simulink model "P8lototoV3p2b"  (R2020b)
settings: Solver=ode5  StartTime=0.0  StopTime=inf  RelTol=1e-3
undefined symbols (not defined in the file): National_Instruments, PCI
libraries: sldrtlib x2, cstblocks x2, simulink x2, pid_lib x1
settings Model: SimulationMode=external  Creator=Usuario_UMA  LastModifiedBy=alumnoic03
settings RTWCC: Description=Simulink Desktop Real-Time  SystemTargetFile=sldrt.tlc  TemplateMakefile=sldrt.tmf  RTWCompilerOptimization=on
settings CodeAppCC: MaxIdLength=95
settings SimulinkDesktopRealTimeCC: TargetPreCompLibLocation=C:\Program Files\MATLAB\R2020\toolbox\sldrt\lib\win64

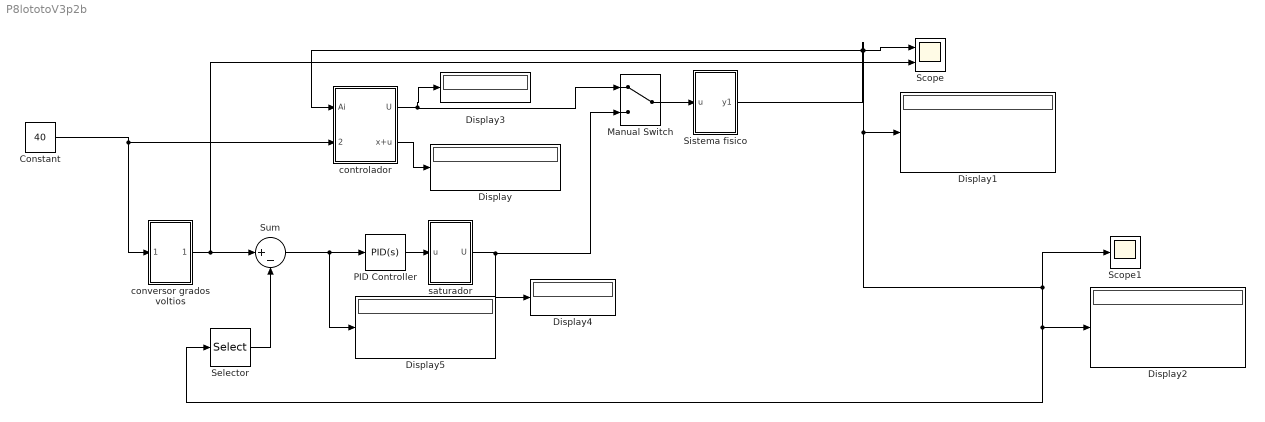
== system P8lototoV3p2b ==
  Constant : Constant  Value=40
  Display{,1..5} (6 alike) : Display
  Manual Switch : ManualSwitch
  PID Controller : pid_lib/PID Controller  Controller=PID  Form=Parallel  TimeDomain=Continuous-time  UseExternalTs=off  SampleTime=-1  IntegratorMethod=Forward Euler  FilterMethod=Forward Euler  ControllerParametersSource=internal  P=1.17  I=1.96  D=0.118  UseFilter=on  N=100  TunerSelectOption=Transfer Function Based (PID Tuner App)  InitialConditionSource=internal  InitialConditionForIntegrator=0  InitialConditionForFilter=0  DifferentiatorICPrevScaledInput=0  ExternalReset=none  TrackingMode=off  Kt=1  LimitOutput=off  SatLimitsSource=internal  UpperSaturationLimit=inf  LowerSaturationLimit=-inf  LinearizeAsGain=on  AntiWindupMode=none  Kb=1  POutMin=[]  POutMax=[]  IOutMin=[]  IOutMax=[]  DOutMin=[]  DOutMax=[]  NOutMin=[]  NOutMax=[]  SumOutMin=[]  SumOutMax=[]  SaturationOutMin=[]  SaturationOutMax=[]  PParamMin=[]  PParamMax=[]  IParamMin=[]  IParamMax=[]  DParamMin=[]  DParamMax=[]  NParamMin=[]  NParamMax=[]  KbParamMin=[]  KbParamMax=[]  KtParamMin=[]  KtParamMax=[]  KbOutMin=[]  KbOutMax=[]  KtOutMin=[]  KtOutMax=[]  IntegratorOutMin=[]  IntegratorOutMax=[]  FilterOutMin=[]  FilterOutMax=[]  SumI1OutMin=[]  SumI1OutMax=[]  SumI2OutMin=[]  SumI2OutMax=[]  SumI3OutMin=[]  SumI3OutMax=[]  SumI4OutMin=[]  SumI4OutMax=[]  SumDOutMin=[]  SumDOutMax=[]  DifferentiatorOutMin=[]  DifferentiatorOutMax=[]  FilterDiffOutCoefMin=[]  FilterDiffOutCoefMax=[]  ReciprocalOutMin=[]  ReciprocalOutMax=[]  SumDenOutMin=[]  SumDenOutMax=[]  SumNumOutMin=[]  SumNumOutMax=[]  DivideOutMin=[]  DivideOutMax=[]  UdiffTsProdOutMin=[]  UdiffTsProdOutMax=[]  NTsProdOutMin=[]  NTsProdOutMax=[]  UintegralTsProdOutMin=[]  UintegralTsProdOutMax=[]  UngainTsProdOutMin=[]  UngainTsProdOutMax=[]  IntegratorContinuousStateAttributes=''  IntegratorStateMustResolveToSignalObject=off  IntegratorRTWStateStorageClass=Auto  FilterContinuousStateAttributes=''  FilterStateMustResolveToSignalObject=off  FilterRTWStateStorageClass=Auto  ParallelPVariant=InternalParameters  IdealPVariant=Disabled  IVariant=InternalParameters  DVariant=InternalParameters  IntegratorVariant=Continuous  SatVariant=Disabled  AWVariant=Passthrough  PCopyVariant=Disabled  TRVariant=Disabled  FdbkBlocksVariant=Forward  IdealPFdbkVariant=Disabled  SatFdbkVariant=Disabled  DerivativeFilterVariant=ContFilter  NVariant=InternalParameters  NCopyVariant=Disabled  FilterICVariant=InternalICsFilter  IntegratorICVariant=InternalICs  ExternalResetVariant=Disabled  TRSumVariant=Passthrough  SumFdbkVariant=Disabled  SumVariant=Sum_PID  TsampFilterVariant=InternalTs  TsampNgainVariant=Passthrough  TsampIntegralVariant=Passthrough  ExternalSaturationOutDataTypeStr=Inherit: Same as second input
  Scope : Scope  NumInputPorts=2
  Scope1 : Scope
  Selector : Selector  InputPortWidth=2  IndexOptions=Index vector (dialog)  Indices=[1]  OutputSizes=1
  Sistema fisico : Subsystem
  Sum : Sum  Inputs=|+-
  controlador : Subsystem
  "conversor grados voltios " : Subsystem  mask{a=4.95, b=0.869}
  saturador : Subsystem
  wires:
  Constant/1 -> "conversor grados voltios "/1(In1), controlador/2(Posicion)
  controlador/2(x+u) -> Display/1
  Sistema fisico/1(y1) -> Selector/1, Display2/1, Scope1/1, Display1/1, Scope/1, controlador/1(Ai)
  Sum/1 -> Display5/1, PID Controller/1
  "conversor grados voltios "/1(Out1) -> Scope/2, Sum/1
  PID Controller/1 -> saturador/1(u)
  Selector/1 -> Sum/2
  controlador/1(U) -> Display3/1, Manual Switch/1
  Manual Switch/1 -> Sistema fisico/1(u)
  saturador/1(U) -> Manual Switch/2, Display4/1

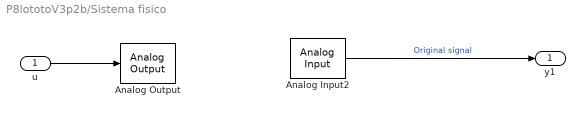
== system P8lototoV3p2b/Sistema fisico ==
  u : Inport
  Analog Input2 : sldrtlib/Analog Input  SampleTime=0.001  MaxMissedTicks=10  ShowMissedTicks=off  YieldWhenWaiting=off  DrvName=National_Instruments/PCI-6014  DrvAddress=4294967295  DrvOptions=[2 0 0 0 0 0]  Channels=[1,2]  RangeMode=1  VoltRange=1  DataType=1
      settings: AttributesFormatString=National Instruments\nPCI-6014 [auto]
  Analog Output : sldrtlib/Analog Output  SampleTime=0.001  MaxMissedTicks=10  ShowMissedTicks=off  YieldWhenWaiting=off  DrvName=National_Instruments/PCI-6014  DrvAddress=4294967295  DrvOptions=[2 0 0 0 0 0]  Channels=1  RangeMode=1  VoltRange=1  InitialValue=[]  FinalValue=[]
      settings: AttributesFormatString=National Instruments\nPCI-6014 [auto]
  y1 : Outport
  wires:
  u/1 -> Analog Output/1
  Analog Input2/1 -> y1/1  "Original signal"

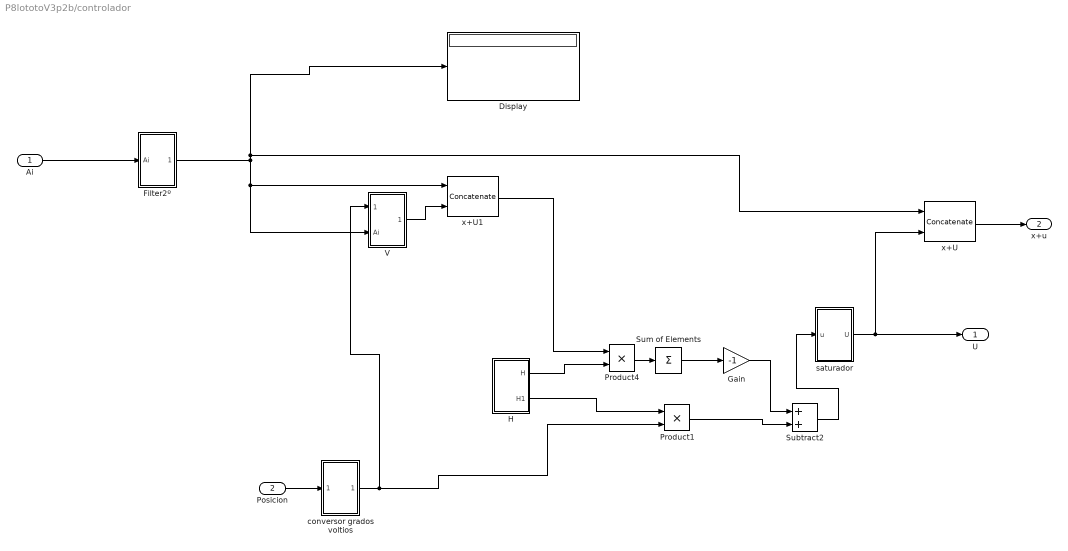
== system P8lototoV3p2b/controlador ==
  Ai : Inport  OutDataTypeStr=double
  Posicion : Inport  Port=2
  Display : Display
  Filter2º : Subsystem
  Gain : Gain  Gain=-1
  H : Subsystem  mask{h1=32.89, h2=1.059, h3=-0.0636}
  Product1 : Product
  Product4 : Product
  Subtract2 : Sum  OutDataTypeStr=double
  Sum of Elements : Sum  Inputs=+
  V : Subsystem
  "conversor grados voltios " : Subsystem  mask{a=4.95, b=0.869}
  saturador : Subsystem
  x+U : Concatenate  ConcatenateDimension=2
  x+U1 : Concatenate  ConcatenateDimension=2
  U : Outport  OutDataTypeStr=double
  x+u : Outport  Port=2
  wires:
  Product4/1 -> Sum of Elements/1
  Gain/1 -> Subtract2/1
  "conversor grados voltios "/1(Out1) -> V/1(In2), Product1/2
  H/1(H) -> Product4/2
  Subtract2/1 -> saturador/1(u)
  H/2(H1) -> Product1/1
  Sum of Elements/1 -> Gain/1
  Product1/1 -> Subtract2/2
  saturador/1(U) -> U/1, x+U/2
  Posicion/1 -> "conversor grados voltios "/1(In1)
  x+U/1 -> x+u/1
  Ai/1 -> Filter2º/1(Ai)
  V/1(Out1) -> x+U1/2
  x+U1/1 -> Product4/1
  Filter2º/1(Out1) -> Display/1, x+U/1, V/2(Ai), x+U1/1

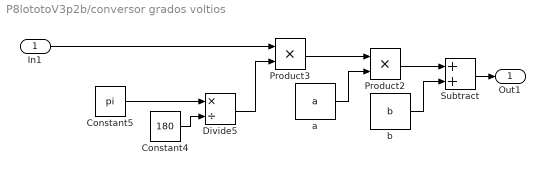
== system P8lototoV3p2b/conversor grados voltios  ==
  In1 : Inport
  Constant4 : Constant  Value=180
  Constant5 : Constant  Value=pi
  Divide5 : Product  Inputs=*/
  Product2 : Product
  Product3 : Product
  Subtract : Sum
  a : Constant  Value=a
  b : Constant  Value=b
  Out1 : Outport
  wires:
  b/1 -> Subtract/2
  Product3/1 -> Product2/1
  Constant4/1 -> Divide5/2
  In1/1 -> Product3/1
  Product2/1 -> Subtract/1
  a/1 -> Product2/2
  Constant5/1 -> Divide5/1
  Divide5/1 -> Product3/2
  Subtract/1 -> Out1/1

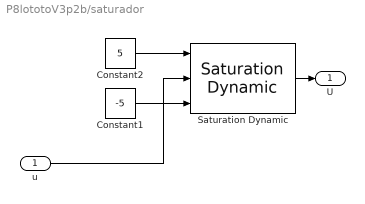
== system P8lototoV3p2b/saturador ==
  u : Inport  OutDataTypeStr=double
  Constant1 : Constant  Value=-5
  Constant2 : Constant  Value=5
  Saturation Dynamic : simulink/Discontinuities/Saturation Dynamic  OutMin=-5  OutMax=5  OutDataTypeStr=Inherit: Same as second input  OutDataType=fixdt(1, 16)  OutScaling=2^-10  DoSatur=off
  U : Outport  OutDataTypeStr=double
  wires:
  u/1 -> Saturation Dynamic/2
  Constant2/1 -> Saturation Dynamic/1
  Saturation Dynamic/1 -> U/1
  Constant1/1 -> Saturation Dynamic/3

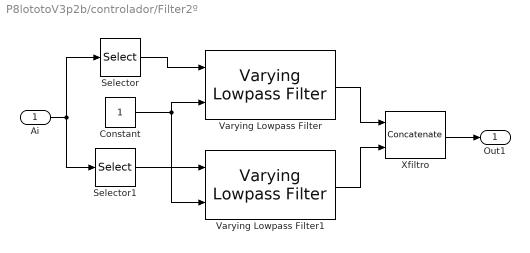
== system P8lototoV3p2b/controlador/Filter2º ==
  Ai : Inport
  Constant : Constant
  Selector : Selector  InputPortWidth=2  IndexOptions=Index vector (dialog)  Indices=[1]  OutputSizes=1
  Selector1 : Selector  InputPortWidth=2  IndexOptions=Index vector (dialog)  Indices=[2]  OutputSizes=1
  Varying Lowpass Filter : cstblocks/Linear Parameter Varying/Varying Lowpass Filter  N=1
  Varying Lowpass Filter1 : cstblocks/Linear Parameter Varying/Varying Lowpass Filter  N=2
  Xfiltro : Concatenate  ConcatenateDimension=2
  Out1 : Outport
  wires:
  Xfiltro/1 -> Out1/1
  Selector/1 -> Varying Lowpass Filter/1
  Varying Lowpass Filter1/1 -> Xfiltro/2
  Selector1/1 -> Varying Lowpass Filter1/1
  Ai/1 -> Selector1/1, Selector/1
  Varying Lowpass Filter/1 -> Xfiltro/1
  Constant/1 -> Varying Lowpass Filter1/2, Varying Lowpass Filter/2

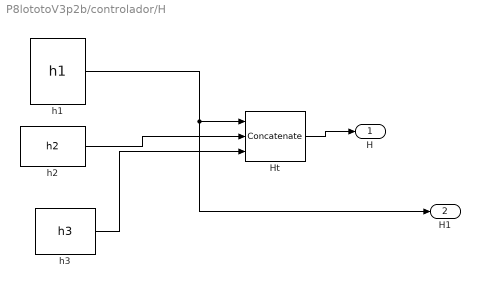
== system P8lototoV3p2b/controlador/H ==
  Ht : Concatenate  NumInputs=3  ConcatenateDimension=2
  h1 : Constant  Value=h1
  h2 : Constant  Value=h2
  h3 : Constant  Value=h3
  H : Outport
  H1 : Outport  Port=2
  wires:
  h1/1 -> H1/1, Ht/1
  h2/1 -> Ht/2
  Ht/1 -> H/1
  h3/1 -> Ht/3

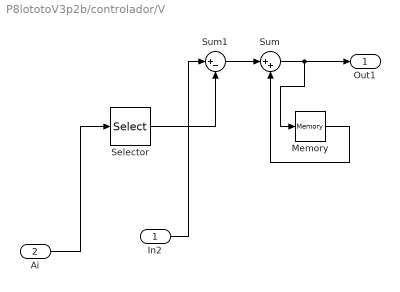
== system P8lototoV3p2b/controlador/V ==
  In2 : Inport
  Ai : Inport  Port=2  PortDimensions=2
  Memory : Memory  InheritSampleTime=on  LinearizeAsDelay=on
  Selector : Selector  InputPortWidth=2  IndexOptions=Index vector (dialog)  Indices=[1]  OutputSizes=1
  Sum : Sum  Inputs=|++
  Sum1 : Sum  Inputs=|+-
  Out1 : Outport
  wires:
  In2/1 -> Sum1/1
  Sum/1 -> Out1/1, Memory/1
  Sum1/1 -> Sum/1
  Memory/1 -> Sum/2
  Ai/1 -> Selector/1
  Selector/1 -> Sum1/2

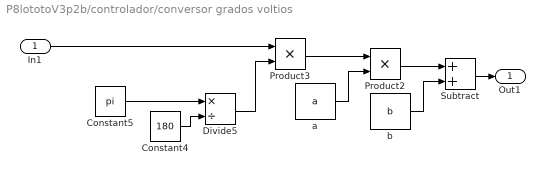
== system P8lototoV3p2b/controlador/conversor grados voltios  ==
  In1 : Inport
  Constant4 : Constant  Value=180
  Constant5 : Constant  Value=pi
  Divide5 : Product  Inputs=*/
  Product2 : Product
  Product3 : Product
  Subtract : Sum
  a : Constant  Value=a
  b : Constant  Value=b
  Out1 : Outport
  wires:
  b/1 -> Subtract/2
  Product3/1 -> Product2/1
  Constant4/1 -> Divide5/2
  In1/1 -> Product3/1
  Product2/1 -> Subtract/1
  a/1 -> Product2/2
  Constant5/1 -> Divide5/1
  Divide5/1 -> Product3/2
  Subtract/1 -> Out1/1

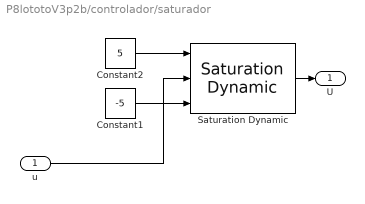
== system P8lototoV3p2b/controlador/saturador ==
  u : Inport  OutDataTypeStr=double
  Constant1 : Constant  Value=-5
  Constant2 : Constant  Value=5
  Saturation Dynamic : simulink/Discontinuities/Saturation Dynamic  OutMin=-5  OutMax=5  OutDataTypeStr=Inherit: Same as second input  OutDataType=fixdt(1, 16)  OutScaling=2^-10  DoSatur=off
  U : Outport  OutDataTypeStr=double
  wires:
  u/1 -> Saturation Dynamic/2
  Constant2/1 -> Saturation Dynamic/1
  Saturation Dynamic/1 -> U/1
  Constant1/1 -> Saturation Dynamic/3
